simulink model "Integration2022b_May06"  (R2022b)
settings: Solver=FixedStepAuto  StartTime=0.0  StopTime=inf  RelTol=1e-3
model workspace (MAT data in the model file):
  L = 4.165
  SL_ROS_VariableLengthArrays_MaxSizes : object (value not decoded)
  finalint = 0
  firstWarning = 1
  originalScenarioChecksum = '114339432DE22364D47BB28FC96DC10C'
values from neighbouring files (symbols this model uses):
  D = cross(B-A,C-A)    [HelperCalculateEgoRefPathInfo.m]
  data =     [Part_of_MCity.mat]    (also in curvedroad_Bhanu.mat; plotWPScript.m = [data, [out.x.Data(:, :, i); out.y.Data(:, :, i)]])
  x = [Vertices(Na,1) Vertices(:,1) Vertices(Nb,1)]    [HelperCalculateEgoRefPathInfo.m]    (also in HelperConvertDSPoseToSim3D.m = actor(1).Position(1); xpts.mat = [-29.9023190589 -34.2715935353 -19.4160603154 -19.4160603154)
  y = [Vertices(Na,2) Vertices(:,2) Vertices(Nb,2)]    [HelperCalculateEgoRefPathInfo.m]    (also in HelperConvertDSPoseToSim3D.m = actor(1).Position(2); VehicleOutputFcn.m = [x(1);x(2); x(3); x(4); x(5);x(6)]; ypts.mat = [-62.3254015256 -62.9079714558 -51.8391427821 -48.6350081661)
  z = zeros(1, length(interpX))    [HelperCalculateEgoRefPathInfo.m]
undefined symbols (not defined in the file or in its folder): MinVelocity, WB
libraries: ros2lib x13, mpcsigdimcheck_private x10, robotalgslib x1, mpclib x1, drivingvehiclecontroller x1, slpidlib x1
(part 5 of 5)

== matlab function Integration2022b_May06/Reference waypoints ==
  data: waypoints output
function waypoints = fcn()


waypoints = [39.99806227837	-83.03238507155	229
39.99806225176	-83.03238507514	229
39.9980622151	-83.03238507952	229
39.99806216774	-83.03238508483	229
39.99806210916	-83.0323850914	229
39.9980620386	-83.03238509932	229
39.99806195496	-83.03238510834	229
39.99806185794	-83.03238511771	229
39.99806174741	-83.03238512699	229
39.99806162342	-83.03238513722	229
39.99806148606	-83.03238514889	229
39.9980613351	-83.03238516134	229
39.99806117106	-83.03238517433	229
39.99806099373	-83.03238518809	229
39.99806080287	-83.03238520311	229
39.99806059877	-83.03238521974	229
39.9980603816	-83.03238523758	229
39.99806015088	-83.03238525624	229
39.99805990597	-83.03238527514	229
39.99805964671	-83.03238529435	229
39.99805937279	-83.03238531348	229
39.99805908445	-83.03238533236	229
39.99805878124	-83.03238535135	229
39.99805846301	-83.0323853721	229
39.99805813043	-83.03238539447	229
39.99805778345	-83.03238541821	229
39.99805742217	-83.03238544562	229
39.99805704525	-83.03238547719	229
39.99805665066	-83.03238551184	229
39.99805623779	-83.03238554698	229
39.99805580651	-83.03238558132	229
39.99805535566	-83.03238561318	229
39.99805488245	-83.03238564368	229
39.99805438579	-83.0323856757	229
39.99805386398	-83.03238570799	229
39.99805331699	-83.03238573957	229
39.99805274668	-83.03238577085	229
39.99805215422	-83.03238580623	229
39.99805153901	-83.03238584858	229
39.99805090072	-83.03238589397	229
39.99805023847	-83.03238593501	229
39.99804955387	-83.0323859732	229
39.99804884854	-83.03238600929	229
39.99804812134	-83.03238604341	229
39.99804736942	-83.03238607335	229
39.99804659222	-83.03238609894	229
39.99804579135	-83.03238612215	229
39.99804496763	-83.0323861475	229
39.99804412175	-83.03238617519	229
39.99804325484	-83.03238620332	229
39.99804236657	-83.032386228	229
39.99804145321	-83.03238625152	229
39.99804051343	-83.032386277	229
39.99803954941	-83.03238630202	229
39.9980385642	-83.03238632304	229
39.9980375606	-83.03238633651	229
39.99803653652	-83.03238634697	229
39.99803548964	-83.03238635868	229
39.99803442351	-83.03238637053	229
39.9980333402	-83.03238638456	229
39.99803223852	-83.03238640484	229
39.99803111484	-83.03238642781	229
39.99802996541	-83.0323864486	229
39.99802879006	-83.03238647172	229
39.99802759101	-83.03238649686	229
39.99802637196	-83.03238652146	229
39.99802513502	-83.03238654417	229
39.99802387934	-83.03238656564	229
39.99802260234	-83.032386585	229
39.99802130181	-83.03238660287	229
39.99801998372	-83.03238661609	229
39.99801864897	-83.0323866234	229
39.99801729425	-83.03238662973	229
39.99801591803	-83.03238663905	229
39.99801452252	-83.03238665271	229
39.99801311009	-83.03238666735	229
39.99801167682	-83.03238667923	229
39.99801021795	-83.03238668921	229
39.99800873742	-83.03238671672	229
39.99800724147	-83.03238675343	229
39.9980057318	-83.03238678991	229
39.99800420585	-83.03238682836	229
39.99800266269	-83.03238687154	229
39.99800110662	-83.032386922	229
39.99799954247	-83.03238697846	229
39.99799796658	-83.03238703209	229
39.99799637829	-83.03238708819	229
39.99799477883	-83.03238714956	229
39.99799317104	-83.0323872162	229
39.99799155708	-83.03238728636	229
39.99798993813	-83.03238735626	229
39.99798831859	-83.03238743124	229
39.99798670493	-83.03238751066	229
39.99798509358	-83.03238761542	229
39.9979834807	-83.0323877503	229
39.99798186778	-83.03238789974	229
39.99798025748	-83.03238805807	229
39.99797865179	-83.03238822672	229
39.99797704903	-83.03238840551	229
39.99797544282	-83.03238859589	229
39.99797383264	-83.03238880248	229
39.99797222769	-83.03238902288	229
39.99797062788	-83.03238924809	229
39.9979690293	-83.03238948477	229
39.99796743185	-83.03238974006	229
39.99796583588	-83.0323900133	229
39.9979642362	-83.03239029449	229
39.99796263389	-83.03239057328	229
39.99796103244	-83.0323908433	229
39.99795942781	-83.03239109745	229
39.99795781729	-83.03239132289	229
39.99795620105	-83.03239152875	229
39.99795457923	-83.03239173027	229
39.99795295492	-83.03239193247	229
39.99795132891	-83.03239214768	229
39.99794969932	-83.03239238496	229
39.99794806376	-83.03239264698	229
39.99794642222	-83.03239292936	229
39.99794478006	-83.03239322594	229
39.99794313768	-83.03239353257	229
39.9979414933	-83.03239384218	229
39.99793984742	-83.03239414331	229
39.99793819886	-83.03239443095	229
39.99793655178	-83.03239470689	229
39.99793491169	-83.03239496597	229
39.99793327721	-83.03239520892	229
39.99793165059	-83.03239545168	229
39.9979300343	-83.03239571043	229
39.99792842977	-83.0323959992	229
39.99792683979	-83.03239632589	229
39.9979252643	-83.03239668805	229
39.99792370386	-83.03239708278	229
39.99792216401	-83.03239751642	229
39.9979206462	-83.0323979888	229
39.99791914359	-83.03239848642	229
39.99791764595	-83.03239900233	229
39.99791615186	-83.03239953319	229
39.99791466259	-83.03240007282	229
39.99791317524	-83.03240062214	229
39.99791169074	-83.03240118781	229
39.99791021889	-83.0324017789	229
39.99790876832	-83.03240240037	229
39.99790734031	-83.03240305497	229
39.9979059366	-83.03240375108	229
39.99790455697	-83.03240449129	229
39.99790319965	-83.03240526838	229
39.9979018623	-83.03240607819	229
39.99790054388	-83.0324069275	229
39.99789924017	-83.03240780389	229
39.99789795049	-83.0324086981	229
39.99789667841	-83.03240961142	229
39.99789542324	-83.03241054286	229
39.99789418065	-83.03241147988	229
39.99789295424	-83.03241244086	229
39.99789174752	-83.03241344165	229
39.99789056469	-83.03241449101	229
39.99788941669	-83.03241558983	229
39.99788830671	-83.03241672758	229
39.99788723077	-83.03241790049	229
39.99788618145	-83.0324191005	229
39.99788515923	-83.0324203259	229
39.99788416924	-83.03242157149	229
39.99788321561	-83.03242283345	229
39.99788229438	-83.03242411282	229
39.99788140433	-83.03242541542	229
39.99788054065	-83.03242674735	229
39.99787969403	-83.03242809984	229
39.99787885465	-83.03242946278	229
39.99787802132	-83.03243083544	229
39.9978772039	-83.03243222385	229
39.99787641925	-83.03243363939	229
39.99787567528	-83.03243508332	229
39.99787496988	-83.0324365466	229
39.99787429569	-83.03243802253	229
39.99787365269	-83.0324395127	229
39.99787304377	-83.03244102356	229
39.99787246485	-83.03244254724	229
39.99787190846	-83.03244407586	229
39.99787137491	-83.03244561086	229
39.99787086386	-83.03244715503	229
39.99787037513	-83.0324487089	229
39.99786991211	-83.03245027402	229
39.99786948354	-83.03245185647	229
39.99786908916	-83.03245345588	229
39.99786871729	-83.03245506829	229
39.9978683647	-83.03245669359	229
39.99786803715	-83.03245833968	229
39.99786773632	-83.03246000806	229
39.99786745744	-83.03246169633	229
39.99786719281	-83.03246340902	229
39.99786693468	-83.03246514706	229
39.99786667599	-83.03246690344	229
39.99786642418	-83.0324686747	229
39.99786618854	-83.03247046119	229
39.99786597319	-83.03247226404	229
39.99786577648	-83.03247408263	229
39.99786560434	-83.03247591964	229
39.99786546061	-83.032477773	229
39.99786534078	-83.03247964459	229
39.99786523319	-83.03248153436	229
39.99786513581	-83.03248343819	229
39.99786504837	-83.03248535536	229
39.99786496749	-83.03248728907	229
39.99786489365	-83.03248923904	229
39.99786481994	-83.03249120448	229
39.99786474423	-83.03249318412	229
39.99786466911	-83.03249517904	229
39.99786459377	-83.032497197	229
39.99786452542	-83.0324992391	229
39.99786447127	-83.03250130323	229
39.99786442322	-83.03250339124	229
39.99786438645	-83.03250549842	229
39.9978643631	-83.03250762136	229
39.99786434627	-83.03250976231	229
39.99786433688	-83.03251192181	229
39.99786434016	-83.03251409964	229
39.99786434669	-83.03251629877	229
39.99786434583	-83.03251852022	229
39.99786434043	-83.03252076373	229
39.99786433301	-83.03252303071	229
39.99786432779	-83.03252532379	229
39.99786432048	-83.03252763963	229
39.99786431669	-83.03252997945	229
39.997864317	-83.03253234028	229
39.99786432461	-83.0325347215	229
39.99786434027	-83.03253712725	229
39.99786436092	-83.03253955137	229
39.9978643841	-83.03254198813	229
39.99786441753	-83.03254444361	229
39.99786445547	-83.03254692468	229
39.99786448592	-83.03254943286	229
39.99786451891	-83.0325519629	229
39.99786455985	-83.03255451664	229
39.99786460762	-83.03255709063	229
39.99786465578	-83.0325596824	229
39.99786470253	-83.03256229242	229
39.99786474797	-83.03256492016	229
39.997864797	-83.03256756004	229
39.99786485285	-83.03257022124	229
39.99786491758	-83.0325729155	229
39.99786499063	-83.03257563502	229
39.99786506073	-83.03257836953	229
39.99786513394	-83.03258112215	229
39.9978652298	-83.03258389599	229
39.99786534595	-83.0325866869	229
39.99786547643	-83.03258949686	229
39.99786561573	-83.032592323	229
39.99786575889	-83.03259517057	229
39.99786589239	-83.03259804605	229
39.99786601256	-83.03260094921	229
39.99786613481	-83.03260387184	229
39.99786625483	-83.03260680408	229
39.99786635896	-83.03260975523	229
39.99786645982	-83.03261271915	229
39.99786657963	-83.03261569892	229
39.99786672562	-83.03261870432	229
39.99786688394	-83.03262173864	229
39.99786705237	-83.03262480073	229
39.99786722844	-83.0326278868	229
39.99786740788	-83.03263099097	229
39.99786758359	-83.03263411042	229
39.99786774092	-83.03263724999	229
39.99786788269	-83.03264040506	229
39.99786802862	-83.03264358187	229
39.99786817869	-83.03264677913	229
39.99786832599	-83.03264999752	229
39.99786847337	-83.03265323294	229
39.99786861926	-83.03265648672	229
39.99786876618	-83.03265976261	229
39.99786891796	-83.03266304875	229
39.99786907453	-83.03266635107	229
39.99786921381	-83.03266967574	229
39.99786935201	-83.03267301512	229
39.9978694976	-83.0326763637	229
39.99786963936	-83.0326797353	229
39.99786978159	-83.0326831261	229
39.99786992807	-83.03268653581	229
39.99787008286	-83.03268995689	229
39.99787024115	-83.0326933889	229
39.99787040459	-83.03269682899	229
39.99787055911	-83.03270026596	229
39.99787070335	-83.03270370666	229
39.99787083062	-83.03270716806	229
39.99787095456	-83.03271064687	229
39.99787108721	-83.032714143	229
39.99787122055	-83.03271764414	229
39.99787135709	-83.03272115129	229
39.99787150799	-83.03272465537	229
39.99787167344	-83.03272815331	229
39.99787184525	-83.03273164835	229
39.99787201876	-83.03273514223	229
39.99787218578	-83.03273863322	229
39.99787234887	-83.03274212339	229
39.997872507	-83.03274560955	229
39.99787265469	-83.03274909034	229
39.9978727989	-83.03275256377	229
39.99787294196	-83.03275603359	229
39.99787308996	-83.03275949873	229
39.99787325072	-83.03276295828	229
39.99787341699	-83.03276641961	229
39.99787359031	-83.03276988277	229
39.9978737753	-83.03277334356	229
39.99787395547	-83.0327767968	229
39.99787412922	-83.0327802426	229
39.99787430473	-83.032783686	229
39.99787447268	-83.03278712923	229
39.99787463889	-83.03279058106	229
39.99787481081	-83.03279403758	229
39.99787498137	-83.03279749736	229
39.99787513555	-83.03280095616	229
39.99787529897	-83.03280441157	229
39.99787547253	-83.0328078565	229
39.99787564259	-83.03281129366	229
39.99787581239	-83.03281472407	229
39.99787598214	-83.03281815266	229
39.99787615917	-83.03282157991	229
39.99787633443	-83.03282501003	229
39.997876504	-83.03282844137	229
39.99787665183	-83.03283187843	229
39.99787678621	-83.0328353223	229
39.99787690553	-83.03283877621	229
39.99787700362	-83.03284224674	229
39.99787710454	-83.03284570243	229
39.99787722889	-83.03284914005	229
39.99787737277	-83.03285256078	229
39.99787754622	-83.03285593517	229
39.99787775435	-83.03285926456	229
39.99787796498	-83.03286256525	229
39.99787815027	-83.0328658544	229
39.99787829223	-83.03286915045	229
39.99787838531	-83.03287245045	229
39.99787846441	-83.03287576495	229
39.99787855093	-83.03287909401	229
39.99787865153	-83.0328824333	229
39.99787877206	-83.03288578091	229
39.99787892839	-83.03288914376	229
39.99787910768	-83.03289251268	229
39.99787928706	-83.03289586935	229
39.99787945725	-83.03289919619	229
39.99787961115	-83.03290248163	229
39.99787975154	-83.03290573283	229
39.99787988006	-83.03290895257	229
39.99787999759	-83.03291214074	229
39.99788010287	-83.03291530282	229
39.99788020246	-83.03291844707	229
39.99788031008	-83.03292157926	229
39.99788042845	-83.03292469795	229
39.99788055421	-83.0329278056	229
39.99788067857	-83.03293090416	229
39.99788079995	-83.03293399092	229
39.99788091585	-83.03293705914	229
39.99788101887	-83.03294010748	229
39.99788111836	-83.03294314065	229
39.9978812164	-83.03294615374	229
39.99788131507	-83.03294914031	229
39.99788141671	-83.03295209899	229
39.99788152354	-83.03295502836	229
39.99788163122	-83.03295793483	229
39.99788173483	-83.032960824	229
39.99788183171	-83.03296369253	229
39.99788192688	-83.03296654083	229
39.99788202155	-83.03296937561	229
39.99788211019	-83.03297219477	229
39.99788219431	-83.03297499566	229
39.99788226936	-83.03297778492	229
39.99788234711	-83.03298055729	229
39.9978824267	-83.03298330655	229
39.99788251289	-83.03298604418	229
39.99788260383	-83.03298876948	229
39.99788269838	-83.0329914781	229
39.99788279279	-83.03299417311	229
39.99788289181	-83.03299685754	229
39.99788299047	-83.03299953561	229
39.99788309464	-83.03300220289	229
39.99788319067	-83.03300485837	229
39.9978832776	-83.0330075037	229
39.9978833531	-83.03301014009	229
39.99788343172	-83.03301277377	229
39.997883523	-83.03301540313	229
39.99788362637	-83.03301802093	229
39.99788373601	-83.03302063038	229
39.99788385289	-83.03302323263	229
39.99788397684	-83.033025826	229
39.99788410322	-83.03302840555	229
39.99788423324	-83.03303096782	229
39.997884379	-83.03303352123	229
39.99788453937	-83.03303606523	229
39.99788472008	-83.0330385988	229
39.99788491352	-83.03304111978	229
39.99788511572	-83.03304362706	229
39.99788533631	-83.03304612153	229
39.99788556759	-83.03304860474	229
39.99788580208	-83.03305107576	229
39.99788603797	-83.03305353151	229
39.99788629057	-83.03305596926	229
39.99788656356	-83.03305839293	229
39.99788686596	-83.03306080162	229
39.99788720319	-83.03306318873	229
39.99788758425	-83.03306555317	229
39.99788800982	-83.03306789619	229
39.99788846913	-83.0330702156	229
39.99788895975	-83.03307251081	229
39.9978894882	-83.03307477537	229
39.99789004175	-83.03307701193	229
39.99789060759	-83.03307923302	229
39.99789119466	-83.03308143911	229
39.9978917997	-83.03308362536	229
39.99789243819	-83.03308577779	229
39.99789311697	-83.03308788874	229
39.99789383158	-83.03308996098	229
39.99789457783	-83.03309199336	229
39.99789535756	-83.03309398856	229
39.99789617063	-83.03309594832	229
39.9978970196	-83.03309787437	229
39.99789790716	-83.03309976787	229
39.99789882643	-83.03310163111	229
39.99789977376	-83.03310346361	229
39.99790074766	-83.03310526432	229
39.99790175883	-83.03310702871	229
39.9979028024	-83.03310875305	229
39.99790387562	-83.03311043376	229
39.99790498207	-83.03311206504	229
39.99790611695	-83.03311364802	229
39.9979072728	-83.03311519072	229
39.9979084484	-83.03311669781	229
39.99790965004	-83.03311816486	229
39.99791088374	-83.03311958253	229
39.99791216007	-83.0331209383	229
39.99791346646	-83.03312223556	229
39.99791478227	-83.03312348732	229
39.99791611545	-83.03312470168	229
39.99791745116	-83.03312590125	229
39.99791878187	-83.0331270931	229
39.99792011302	-83.03312827139	229
39.99792146624	-83.03312939094	229
39.99792284792	-83.03313043844	229
39.99792425702	-83.03313142056	229
39.99792568904	-83.03313234607	229
39.99792714764	-83.03313320782	229
39.99792862747	-83.03313400374	229
39.99793012073	-83.03313473745	229
39.99793162302	-83.03313540712	229
39.99793312224	-83.03313604962	229
39.99793461765	-83.03313668502	229
39.99793611013	-83.03313731275	229
39.99793761009	-83.03313792638	229
39.99793912891	-83.03313852162	229
39.99794067563	-83.03313907806	229
39.99794224525	-83.03313958283	229
39.99794383514	-83.03314004622	229
39.99794544827	-83.03314047099	229
39.99794707246	-83.03314085094	229
39.99794869321	-83.03314119155	229
39.99795030586	-83.0331415112	229
39.99795191356	-83.03314180174	229
39.99795352515	-83.03314204385	229
39.99795511898	-83.03314228106	229
39.99795669749	-83.03314252003	229
39.99795826182	-83.033142751	229
39.99795981829	-83.03314295867	229
39.9979613758	-83.03314314034	229
39.99796293535	-83.03314327907	229
39.99796448968	-83.03314338648	229
39.99796602727	-83.03314349013	229
39.99796755029	-83.03314356918	229
39.99796905909	-83.03314361556	229
39.99797055151	-83.0331436331	229
39.99797202415	-83.03314364756	229
39.99797347605	-83.03314366565	229
39.99797490889	-83.03314368198	229
39.99797633098	-83.03314369617	229
39.99797774542	-83.03314370501	229
39.99797916297	-83.03314371415	229
39.99798058096	-83.03314372785	229
39.9979819959	-83.03314374817	229
39.99798340386	-83.03314377176	229
39.99798479788	-83.03314378597	229
39.99798616992	-83.03314377511	229
39.99798751466	-83.03314375547	229
39.99798883262	-83.03314376177	229
39.99799012553	-83.03314378954	229
39.99799139171	-83.03314382108	229
39.99799262865	-83.03314385481	229
39.99799383823	-83.033143895	229
39.99799501962	-83.03314393683	229
39.99799617313	-83.03314397614	229
39.99799729941	-83.03314400955	229
39.99799839507	-83.03314403597	229
39.99799945575	-83.03314405617	229
39.99800047752	-83.03314407131	229
39.99800146156	-83.03314408337	229
39.99800240247	-83.03314408821	229
39.99800329694	-83.03314409118	229
39.99800414483	-83.03314409974	229
39.99800494734	-83.03314410921	229
39.99800570452	-83.03314411545	229
39.99800641557	-83.03314412348	229
39.9980070818	-83.03314413749	229
39.99800770564	-83.03314415248	229
39.99800828855	-83.03314416343	229
39.99800882983	-83.03314417035	229
39.99800932807	-83.03314417893	229
39.99800978142	-83.03314419151	229
39.99801018801	-83.0331442104	229
39.99801054765	-83.03314423429	229
39.99801086001	-83.03314426169	229
39.99801112427	-83.03314429153	229
39.99801133939	-83.0331443232	229
39.99801150532	-83.03314435534	229
39.99801162287	-83.03314438663	229
39.99801169404	-83.03314441058	229
39.99801171667	-83.03314442597	229
39.9980116959	-83.03314443909	229
39.99801165091	-83.03314445196	229
39.99801160284	-83.03314446755	229
39.99801155776	-83.03314448591	229
39.99801151995	-83.03314450432	229
];

== matlab function Integration2022b_May06/BuckeyeLot Origin ==
  data: origin output
function origin = fcn()

origin = [40.01475404518, -83.03091678753, 229];

end

== stateflow chart Integration2022b_May06/Behavioural Planner/Collision Avoidance ==
  state Stop
    en:
    Brake = 1;
  state Start
    en:
    Stuck = 0;
    ACC = 0;
    LaneChangeCmd = 0;
    %VelCmd = CurrentVelCmd;
  state Follow
    en:
    ACC = 1;
    Brake = 0;
  state LaneChange
    en:
    LaneChangeCmd = 1;
  Stop -> Follow : [EgoSpeed<0.1]
  Follow -> Stop [order 4] : [D2O < 20 && EgoSpeed > 2]
  (default) -> Start
  Follow -> LaneChange [order 2] : [LaneAvailable == 1 && Stuck == 1]
  Start -> Follow : [ObjAhead == 1]
  Follow -> Start [order 3] : [ObjAhead == 0]
  LaneChange -> Start : [LaneChanged == 1]
  Follow -> Follow [order 1] : [(EgoSpeed <= MinSpeed) && after(WaitTime,sec)]{Stuck = 1;}
  data: for function_input; seconds function_input; use function_input; rising function_input; and function_input; falling function_input; edge function_input; triggers function_input; to function_input; move function_input; about function_input; Stuck local; ACC output; WaitTime input; ObjAhead input; MinSpeed input; LaneAvailable input; EgoSpeed input; LaneChanged input; LaneChangeCmd output; Brake output; D2O input
  function Hold(for,seconds, use,rising, and, falling, edge, triggers, to, move, about):
    | function Hold(for,seconds, use,rising, and, falling, edge, triggers, to, move, about)

== matlab function Integration2022b_May06/Behavioural Planner/MATLAB Function ==
  data: Waypoints input; distanceToDestination output; CurrentPose input
function distanceToDestination = fcn(Waypoints, CurrentPose)
    destination = [Waypoints(end, 1) Waypoints(end, 2)];
    CurrentPose(2) = - CurrentPose(2);
    distanceToDestination = norm(destination - CurrentPose(1:2)');
end

== matlab function Integration2022b_May06/Perception Pre-Processing/Subsystem/LatLong to XY ==
  data: origin input; RefLL input; RefXY output; RefX output; RefY output
function [RefXY,RefX,RefY]   = XYZenu(origin, RefLL)
%size_points = length(RefLL); %100

%zup = h*ones(size_points, 1); %100x1

%points_new = [RefLL, zup]; 

%latlong_new = points_new; 

%origin_new = latlong_new(1,:)

%origin_new = [origin(1) origin(2) origin(3)]; %1x3

xyz = lla2enu(RefLL, origin,'ellipsoid'); 
RefX = xyz(:,1);
RefY = xyz(:,2);
RefXY = [xyz(:,1) xyz(:,2)];


end

== matlab function Integration2022b_May06/Perception Pre-Processing/Subsystem/Heading conversion ==
  data: CurrPose output; origin input; CurrPosLL input; h input; theta input; CurrPose_Plot output
function [CurrPose, CurrPose_Plot]  = VehicleCurrent(origin, CurrPosLL, h, theta)
zup = h; 
d = double(CurrPosLL(1:2));
lat = double(d(1));
long = double(d(2));

offsetToCenter = 0.762;

CurrPosLatLong = [lat, long];
point_new = [CurrPosLatLong(1), CurrPosLatLong(2), zup];
angle = double(theta);
x_enu = lla2enu(point_new, origin, 'ellipsoid');

head = 90 - angle;
if head < -180
   head = head + 360;
elseif abs(head) == 180
   head = abs(head);
end

x_enuVehicleCenter = x_enu(1) + offsetToCenter*cosd(head);
y_enuVehicleCenter = x_enu(2) + offsetToCenter*sind(head);

CurrPose = [x_enuVehicleCenter y_enuVehicleCenter head];
CurrPose_Plot = [x_enuVehicleCenter y_enuVehicleCenter];

end

== stateflow chart Integration2022b_May06/Behavioural Planner/Behavioural Planner/Chart ==
  settings: updateMethod=DISCRETE  sampleTime=Ts
  state Stationary
    en,du:
    VelCmd = 0;
    CurrentVelCmd = VelCmd;
    Navi = 0;
    Trans = 0;
    StopSim = 0;
    Tgap = 1;
    HoldBrake = 1;
    Braking = 0;
  state Navigation
    state RailCrossing
      state Stop
        en:
        VelCmd = 0;
        Braking = 1;
        CurrentVelCmd = VelCmd;
      state Approaching
        en:
        Braking = 1;
        Tgap = 0;
        Trans = 0;
      state Transition
        en:
        Tgap = 1;
        Trans = 1;
        Braking = 0;
        VelCmd = SceneSpeed;
        CurrentVelCmd = VelCmd;
      state ExitScene
        en:
        ExitFlag = 1;
      (default) -> Navigation.RailCrossing.Approaching
      Navigation.RailCrossing.Approaching -> Navigation.RailCrossing.Stop [order 1] : [D2S <= 6 && (RRCross == 1 || ObjectDist <= TransDist)]
      Navigation.RailCrossing.Transition -> Navigation.RailCrossing.Approaching [order 2] : [ObjectDist <= TransDist]
      Navigation.RailCrossing.Approaching -> Navigation.RailCrossing.Transition [order 3] : [RRCross == 0 && ObjectDist > TransDist && D2S <= 6]
      Navigation.RailCrossing.Stop -> Navigation.RailCrossing.Transition : [RRCross == 0 && ObjectDist > TransDist]
      Navigation.RailCrossing.Approaching -> Navigation.RailCrossing.ExitScene [order 2] : [SceneID ~= 10]
      Navigation.RailCrossing.Transition -> Navigation.RailCrossing.ExitScene [order 1] : [SceneID == 0]
    state RoundAbout
      state Approaching
        en:
        Braking = 1;
        Trans = 0;
        Tgap = 0;
      state Stop
        en:
        VelCmd = 0;
        Braking = 1;
        CurrentVelCmd = VelCmd;
      state ExitScene
        en:
        ExitFlag = 1;
      state Transition
        en:
        Tgap = 1;
        Trans = 1;
        Braking = 0;
        VelCmd = SceneSpeed;
        CurrentVelCmd = VelCmd;
      (default) -> Navigation.RoundAbout.Approaching
      Navigation.RoundAbout.Approaching -> Navigation.RoundAbout.Stop [order 1] : [D2S <= 6]
      Navigation.RoundAbout.Stop -> Navigation.RoundAbout.Transition : [Clear2Go == 1]
      Navigation.RoundAbout.Approaching -> Navigation.RoundAbout.ExitScene [order 2] : [SceneID ~= 9]
      Navigation.RoundAbout.Transition -> Navigation.RoundAbout.ExitScene : [SceneID == 0]
    state DestCheck
      en,du:
      % dest reached?
      (default) -> (junction 47)
      (junction 47) -> (junction 48) [order 1] : [D2D < 2]
      (junction 47) -> (junction 49) [order 2] : {DestReached = 0;}
      (junction 48) -> (junction 50) : {DestReached = 1;}
      (junction 50) -> (junction 49) : {StopSim = 1;}
      (junction 49) -> (junction 51)
    state TrafficLight [commented out]
      note: Yellow light duration is 1s
      state Stop [commented out]
        en:
        Braking = 1;
        VelCmd = 0;
        CurrentVelCmd = VelCmd;
      state Approaching [commented out]
        en:
        Tgap = 0;
        Trans = 0;
        T2S = 0;
        %if TLstate(1,4) == 1
        Braking = 1;
        %else
        % ACC = 0;
        %end
      state DecisionOnYellow [commented out]
        en:
        T2S = D2S/EgoSpeed;
      state Transition [commented out]
        en:
        Trans = 1;
        Braking = 0;
        Tgap = 1;
        VelCmd = SceneSpeed;
        CurrentVelCmd = VelCmd;
      state ExitScene [commented out]
        en:
        ExitFlag = 1;
      DecisionOnYellow -> Navigation.TrafficLight.Approaching [commented out] : [T2S > 1.2]
      (default) -> Navigation.TrafficLight.Approaching [commented out]
      Navigation.TrafficLight.Approaching -> Navigation.TrafficLight.Stop [commented out] : [D2S <= 6]
      Navigation.TrafficLight.Stop -> Navigation.TrafficLight.Transition [commented out] : [TLstate(1,4) == 3 && ObjectDist > TransDist]
      Navigation.TrafficLight.Transition -> Navigation.TrafficLight.Approaching [commented out] : [TLstate(1,4) == 1  || ObjectDist < TransDist]
      Navigation.TrafficLight.Approaching -> Navigation.TrafficLight.Transition [commented out] : [TLstate(1,4) == 3 && ObjectDist > TransDist]
      Navigation.TrafficLight.Approaching -> Navigation.TrafficLight.ExitScene [commented out] : [SceneID ~= 8]
      Navigation.TrafficLight.Transition -> DecisionOnYellow [commented out] : [TLstate(1,4) == 2]
      DecisionOnYellow -> Navigation.TrafficLight.Transition [commented out] : [T2S <= 1.2]
      Navigation.TrafficLight.Transition -> Navigation.TrafficLight.ExitScene [commented out] : [SceneID == 0]
    state Drive
      en :
      HoldBrake = 0;
      VelCmd = RoadSpeed;
      CurrentVelCmd = VelCmd;
      ExitFlag = 0;
    state Go
      en:
      VelCmd = RoadSpeed;
      CurrentVelCmd = VelCmd;
      Trans = 0;
      ExitFlag = 0;
      Braking = 0;
      HoldBrake = 1;
    state StopSign
      state StoptSign4way
        state CheckInt
          du:
          % stopped?
          % ss priority?
        state CheckSS
          % stopped?
          % ss priority?
        state Transition
          en:
          % stay here while trans?!
          % while ~crossedLimitLine of TargetLane
          Trans = 1;
          Braking = 0;
          Tgap = 1;
          VelCmd = SceneSpeed;
          CurrentVelCmd = VelCmd;
        state ExitScene
          en:
          ExitFlag = 1;
        (default) -> Navigation.StopSign.StoptSign4way.CheckSS
        Navigation.StopSign.StoptSign4way.CheckSS -> Navigation.StopSign.StoptSign4way.CheckInt : [EgoSpeed < VelStop]
        Navigation.StopSign.StoptSign4way.CheckInt -> Navigation.StopSign.StoptSign4way.Transition : [egoSSPriority == 1 && Clear2Go == 1]
        Navigation.StopSign.StoptSign4way.Transition -> Navigation.StopSign.StoptSign4way.ExitScene : [SceneID == 0 && after(2,sec)]
      state SStype
        state Approaching
          en:
          %VelCmd = ApproachingSpeed;
          Braking = 1;
          Trans = 0;
          Tgap = 0;
        state Stop
          en:
          VelCmd = 0;
          Braking = 1;
          CurrentVelCmd = VelCmd;
        Navigation.StopSign.SStype.Stop -> 410 [order 1] : [numSS == 4]
        (default) -> Navigation.StopSign.SStype.Approaching
        Navigation.StopSign.SStype.Approaching -> Navigation.StopSign.SStype.Stop : [D2S <= 15]
        Navigation.StopSign.SStype.Stop -> 414 [order 2] : [numSS == 2]
      state StopSign2way
        state CheckInt
          en:
          VelCmd = 0;
          HoldBrake = 1;
          CurrentVelCmd = VelCmd;
        state CheckSS
          % stopped?
          % ss priority?
        state Transition1
          en:
          % stay here while trans?!
          % while ~crossedLimitLine of TargetLane
          Trans = 1;
          Braking = 0;
          HoldBrake = 0;
          Tgap = 1;
          VelCmd = SceneSpeed;
          CurrentVelCmd = VelCmd;
        state ExitScene1
          en:
          ExitFlag = 1;
        (default) -> Navigation.StopSign.StopSign2way.CheckSS
        Navigation.StopSign.StopSign2way.CheckSS -> Navigation.StopSign.StopSign2way.CheckInt : [EgoSpeed < VelStop]
        Navigation.StopSign.StopSign2way.CheckInt -> Transition1 : [egoSSPriority == 1 && ToAClearance == 1 && after(1,sec)]
        Transition1 -> Navigation.StopSign.StopSign2way.CheckInt [order 2] : [ToAClearance == 0]
        Transition1 -> ExitScene1 [order 1] : [SceneID == 0 && egoExit == 1]
      (default) -> SStype
      416 -> StoptSign4way
      411 -> StopSign2way
    Go -> RailCrossing [order 2] : [SceneID == 10]
    Drive -> RailCrossing [order 1] : [SceneID == 10]
    RailCrossing -> Go : [ExitFlag == 1]
    Go -> RoundAbout [order 3] : [SceneID == 9]
    Drive -> RoundAbout [order 2] : [SceneID == 9]
    RoundAbout -> Go : [ExitFlag == 1]
    (default) -> DestCheck
    Drive -> TrafficLight [commented out] : [SceneID == 8]
    DestCheck -> Drive : [DestReached == 0]
    Go -> TrafficLight [commented out] : [SceneID == 8]
    Drive -> DestCheck [order 4] : [D2D < 2]
    TrafficLight -> Go [commented out] : [ExitFlag == 1]
    Drive -> StopSign [order 3] : [SceneID == 7]
    StopSign -> Go : [ExitFlag == 1]
    Go -> DestCheck [order 1] : [SceneID == 0]
    Go -> StopSign [order 4] : [SceneID == 7]
  (default) -> Stationary
  Stationary -> Navigation : [Navigate == 1]
  Navigation -> Stationary : [Navigate == 0 || DestReached == 1]
  data: TLstate input; numSS input; egoExit input; ToAClearance input; TransDist input; ApproachingSpeed input; EgoSpeed input; ObjectDist input; SceneSpeed input; SDist input; RRCross input; D2S input; DestReached local; Navigate input; ExitFlag local; D2D input; Clear2Go input; RoadSpeed input; CurrentVelCmd local; Navi local; VelCmd output; HoldBrake output; SceneID input; Tgap output; Trans output; StopSim output; Braking output; T2S local; VelStop input; egoSSPriority input

== matlab function Integration2022b_May06/Perception Pre-Processing/Object Track A ==
  data: u input; y output; origin input
function y = fcn(u, origin)
if any(u, "all")
    u1 = u(1:693);
    y = double(reshape(u1, 11, 63))';
    height = ones(63, 1) * 229;
    ObjectTrackLL = [y(:, 10), y(:, 11), height];
    ObjectTrackXY =  lla2enu(ObjectTrackLL, origin, 'ellipsoid');                   % Traffic Sign Lat-Long to XY Coordinate Conversion
    y(:, 10) = ObjectTrackXY(:, 1);
    y(:, 11) = ObjectTrackXY(:, 2);
else
    y = double(-1*ones(63, 11));
end

== matlab function Integration2022b_May06/Perception Pre-Processing/Road state ==
  data: u input; y output
function y = fcn(u)
if any(u, "all")
    u1 = u(1:9);
    y = double(reshape(u1, 1, 9));
else
   y = double(-1*ones(1, 9));
end

== matlab function Integration2022b_May06/Perception Pre-Processing/Traffic signs ==
  data: matC input; y output; origin input
function y = fcn(matC, origin)
% if any(u(:, 1), "all")
    u1 = matC(1:441);
    y = double(reshape(u1, 7, 63))';
    height = ones(63, 1) * 229;
    trafficSignLL = [y(:, 6), y(:, 7), height];
    SignXY =  lla2enu(trafficSignLL, origin, 'ellipsoid');                   % Traffic Sign Lat-Long to XY Coordinate Conversion
    y(:, 6) = SignXY(:, 1);
    y(:, 7) = SignXY(:, 2);
 
% else
%    y = double(-1*ones(7, 63))';
end

== matlab function Integration2022b_May06/Perception Pre-Processing/Traffic signals ==
  data: u input; y output; origin input
function y = fcn(u, origin)
if any(u, "all")
    u1 = u(1:1386);
    y = double(reshape(u1, 22, 63))';
    height = ones(63, 1) * 229;
    trafficSignalLL = [y(:, 21), y(:, 22), height];
    SignalXY =  lla2enu(trafficSignalLL, origin, 'ellipsoid');                   % Traffic Sign Lat-Long to XY Coordinate Conversion
    y(:, 21) = SignalXY(:, 1);
    y(:, 22) = SignalXY(:, 2);
else
   y = double(-1*ones(63, 22));
end

== matlab function Integration2022b_May06/Subsystem/Distance to Traffic Sign ==
  data: currentDistanceTravelled input; relativeDistanceToScene output; signLatPose input; signLongPose input; ego_vel input; cumulativeDistance input; CurrentPose input; RefXY input; sceneDistance output; sceneDistance input; signPose output
function [relativeDistanceToScene, sceneDistance,signPose] = fcn(currentDistanceTravelled, signLatPose, signLongPose, ego_vel, cumulativeDistance, CurrentPose, RefXY, sceneDistance)

signPose=[40 40];
if signLatPose ~= -1
    % X front side of car, Y right side of car=

    thetaSS = atan2d(signLongPose, signLatPose);

    
    beta = thetaSS+CurrentPose(3) - 90;
    alphaVector = norm([signLongPose, signLatPose]);
    xSS = alphaVector*cosd(beta);
    ySS = alphaVector*sind(beta);
    signPose = [xSS + CurrentPose(1), ySS + CurrentPose(2)];
    
    %%%
    % signPose = [RefXY(end,1) RefXY(end,2)];

    distance = zeros(length(RefXY),1);
    for j = 1:length(RefXY)
        distance(j) = norm(signPose(1:2) - RefXY(j,1:2));
    end
    
    [~, ind] = mink(distance,2);
    
    if ind(1) > ind(2)
        ind = [ind(2); ind(1)];
    end

    sceneDistance = cumulativeDistance(ind(1));                         % Distance to scene/sign, local origin
    relativeDistanceToScene = sceneDistance - currentDistanceTravelled; % Longitudinal Distance from Ego Vehicle to Scene
    %%%
else
    relativeDistanceToScene = sceneDistance - currentDistanceTravelled;
end

end
